simulink library "ExternalChimeProcess"  (R2022b)
settings: Solver=VariableStepAuto  StartTime=0.0  StopTime=10.0  RelTol=1e-3
libraries: ExternalChimeProcessBtc x1
settings Model: Creator=nikunj.tapodhan  LastModifiedBy=kl13806
settings SolverCC: AlgebraicLoopSolver=TrustRegion
settings DebuggingCC: UnconnectedInputMsg=warning  UnconnectedOutputMsg=warning  UnconnectedLineMsg=warning  SFMachineParentedDataDiag=warning  ArithmeticOperatorsInVariantConditions=warning
settings ModelReferenceCC: EnableRefExpFcnMdlSchedulingChecks=on
settings SFSimCC: CustomCodeUndefinedFunction=UseInterfaceOnly
settings RTWCC: DLArmComputeVersion=19.05

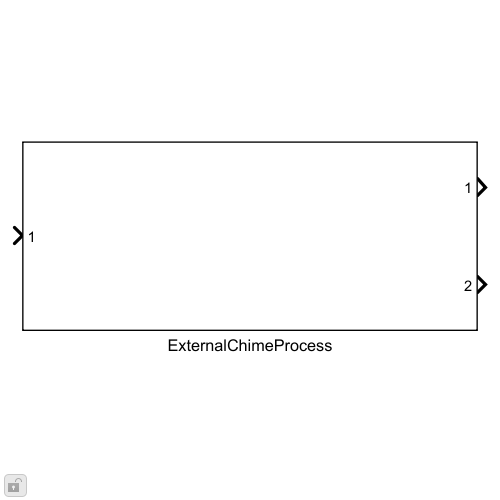
[thumbnail: Simulink's stored preview of the top-level diagram]
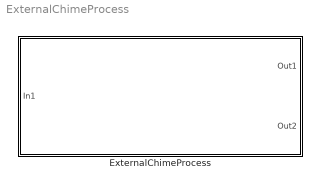
== system ExternalChimeProcess ==
  ExternalChimeProcess : Subsystem  mask{externalChimeCancel=0, frameSize=32, numExtChimes=1}
      mask init:
      | blkh = gcbh;
      | % Copy discrete mask parameters into a classdef object
      | InnerLinkConfig = ExternalChimeProcessConfig;
      | InnerLinkConfig.ExternalChimeCancel = externalChimeCancel;
      | InnerLinkConfig.FrameSize = frameSize;
      | InnerLinkConfig.NumExtChimes = numExtChimes;

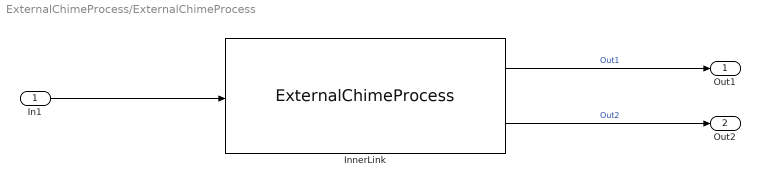
== system ExternalChimeProcess/ExternalChimeProcess ==
  In1 : Inport
  InnerLink : ExternalChimeProcessBtc/ExternalChimeProcess  Config=InnerLinkConfig
      settings: SourceProductName=Bose Blocklib
  Out1 : Outport
  Out2 : Outport  Port=2
  wires:
  InnerLink/1 -> Out1/1  "Out1"
  InnerLink/2 -> Out2/1  "Out2"
  In1/1 -> InnerLink/1
